simulink model "QuadModel"  (R2022b)
settings: Solver=VariableStepAuto  StartTime=0.0  StopTime=50  RelTol=1e-3  AbsTol=1e-3  EnableMultiTasking=on
undefined symbols (not defined in the file): Ixx, Iyy, Izz, k, mass, prD, prI, prP, X, Y, Z, zD, zI, zP
libraries: sm_lib x42, nesl_utility x35, slpidlib x4
(part 1 of 3)
settings Model: Creator=hrishavdas  LastModifiedBy=sudip
settings SolverCC: AutoScaleAbsTol=off  AlgebraicLoopSolver=TrustRegion  MaxZcPerStep=1
settings DataIOCC: LimitDataPoints=on  MaxDataPoints=10000
settings OptimizationCC: LifeSpan=inf
settings DebuggingCC: UnconnectedInputMsg=warning  UnconnectedOutputMsg=warning  UnconnectedLineMsg=warning  AllowSymbolicDim=off  SFUnexpectedBacktrackingDiag=warning  SFNoUnconditionalDefaultTransitionDiag=warning  SFExecutionAtInitializationDiag=none  SFMachineParentedDataDiag=warning  ArithmeticOperatorsInVariantConditions=warning
settings ModelReferenceCC: EnableRefExpFcnMdlSchedulingChecks=on
settings SFSimCC: SimUseLocalCustomCode=off  CustomCodeUndefinedFunction=UseInterfaceOnly
settings RTWCC: RTWUseLocalCustomCode=off  DLArmComputeVersion=19.05
settings CodeAppCC: StateflowObjectComments=on
settings GRTTargetCC: TargetLangStandard=C89/C90 (ANSI)
settings ConfigComp: CovMetricSettings=dw  CovSaveCumulativeToWorkspaceVar=on  CovSaveSingleToWorkspaceVar=on  CovExternalEMLEnable=off  CovSFcnEnable=off
settings SimscapeCC: SimscapeLogType=all  SimscapeLogSimulationStatistics=on  SimscapeLogDataHistory=10000

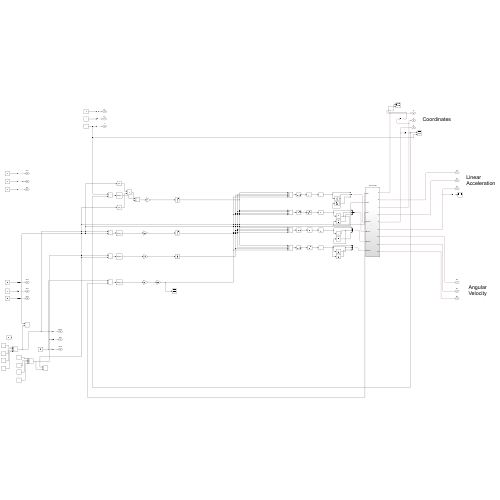
[thumbnail: Simulink's stored preview of the top-level diagram]
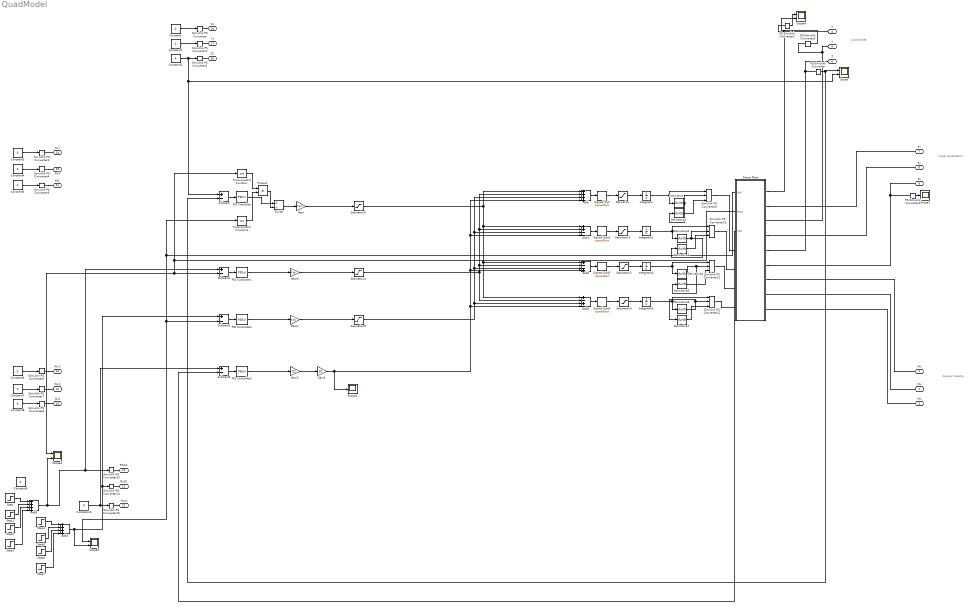
== system QuadModel ==
  note: Coordinates
  note: Linear Acceleration
  note: Angular Velocity
  Add : Sum  Inputs=++++
  Add1 : Sum  Inputs=++--
  Add2 : Sum  Inputs=+--+
  Add3 : Sum  Inputs=+-+-
  Add4 : Sum  Inputs=++++
  Add5 : Sum  Inputs=++++
  Constant{,1,3..9,11} (10 alike) : Constant  Value=0
  Constant2 : Constant  Value=4
  Derivative{,1..7} (8 alike) : Derivative
  Divide : Product  Inputs=*/
  Drone Plant : Subsystem
  Gain : Gain  Gain=mass
  Gain1 : Gain  Gain=Ixx
  Gain2 : Gain  Gain=Izz
  Gain3 : Gain  Gain=10
  Gain6 : Gain  Gain=Iyy
  Integrator{,2,4,6} (4 alike) : Integrator
  PID Controller : slpidlib/PID Controller  Controller=PID  Form=Parallel  TimeDomain=Continuous-time  UseExternalTs=off  SampleTime=-1  IntegratorMethod=Forward Euler  FilterMethod=Forward Euler  ControllerParametersSource=internal  P=zP  I=zI  UseKiTs=off  D=zD  N=100  UseFilter=on  TunerSelectOption=Transfer Function Based (PID Tuner App)  InitialConditionSource=internal  InitialConditionForIntegrator=0  InitialConditionForFilter=0  DifferentiatorICPrevScaledInput=0  ExternalReset=none  TrackingMode=off  Kt=1  LimitOutput=off  SatLimitsSource=internal  UpperSaturationLimit=inf  LowerSaturationLimit=-inf  LinearizeAsGain=on  AntiWindupMode=none  Kb=1  LimitIntegrator=off  UpperIntegratorSaturationLimit=inf  LowerIntegratorSaturationLimit=-inf  POutMin=[]  POutMax=[]  IOutMin=[]  IOutMax=[]  DOutMin=[]  DOutMax=[]  NOutMin=[]  NOutMax=[]  SumOutMin=[]  SumOutMax=[]  SaturationOutMin=[]  SaturationOutMax=[]  PParamMin=[]  PParamMax=[]  IParamMin=[]  IParamMax=[]  DParamMin=[]  DParamMax=[]  NParamMin=[]  NParamMax=[]  KbParamMin=[]  KbParamMax=[]  KtParamMin=[]  KtParamMax=[]  KbOutMin=[]  KbOutMax=[]  KtOutMin=[]  KtOutMax=[]  IntegratorOutMin=[]  IntegratorOutMax=[]  FilterOutMin=[]  FilterOutMax=[]  SumI1OutMin=[]  SumI1OutMax=[]  SumI2OutMin=[]  SumI2OutMax=[]  SumI3OutMin=[]  SumI3OutMax=[]  SumI4OutMin=[]  SumI4OutMax=[]  SumDOutMin=[]  SumDOutMax=[]  DifferentiatorOutMin=[]  DifferentiatorOutMax=[]  FilterDiffOutCoefMin=[]  FilterDiffOutCoefMax=[]  ReciprocalOutMin=[]  ReciprocalOutMax=[]  SumDenOutMin=[]  SumDenOutMax=[]  SumNumOutMin=[]  SumNumOutMax=[]  DivideOutMin=[]  DivideOutMax=[]  UdiffTsProdOutMin=[]  UdiffTsProdOutMax=[]  NTsProdOutMin=[]  NTsProdOutMax=[]  UintegralTsProdOutMin=[]  UintegralTsProdOutMax=[]  UngainTsProdOutMin=[]  UngainTsProdOutMax=[]  ClampingZeroOutDataTypeStr=Inherit: Inherit via back propagation  ClampingZeroOutMin=[]  ClampingZeroOutMax=[]  FilterDenConstantOutDataTypeStr=Inherit: Inherit via back propagation  FilterDenConstantOutMin=[]  FilterDenConstantOutMax=[]  PCopyOutDataTypeStr=Inherit: Inherit via back propagation  PCopyOutMin=[]  PCopyOutMax=[]  NCopyOutDataTypeStr=Inherit: Inherit via back propagation  NCopyOutMin=[]  NCopyOutMax=[]  IntegratorContinuousStateAttributes=''  IntegratorStateMustResolveToSignalObject=off  IntegratorRTWStateStorageClass=Auto  FilterContinuousStateAttributes=''  FilterStateMustResolveToSignalObject=off  FilterRTWStateStorageClass=Auto  ParallelPVariant=InternalParameters  IdealPVariant=Disabled  IVariant=InternalParameters  DVariant=InternalParameters  IntegratorVariant=Continuous  SatVariant=Disabled  AWVariant=Passthrough  PCopyVariant=Disabled  TRVariant=Disabled  FdbkBlocksVariant=Forward  IdealPFdbkVariant=Disabled  SatFdbkVariant=Disabled  DerivativeFilterVariant=ContFilter  NVariant=InternalParameters  NCopyVariant=Disabled  FilterICVariant=InternalICsFilter  IntegratorICVariant=InternalICs  ExternalResetVariant=Disabled  TRSumVariant=Passthrough  SumFdbkVariant=Disabled  SumVariant=Sum_PID  TsampFilterVariant=InternalTs  TsampNgainVariant=Passthrough  TsampIntegralVariant=Passthrough  ExternalSaturationOutDataTypeStr=Inherit: Same as second input
  PID Controller1 : slpidlib/PID Controller  Controller=PID  Form=Parallel  TimeDomain=Continuous-time  UseExternalTs=off  SampleTime=-1  IntegratorMethod=Forward Euler  FilterMethod=Forward Euler  ControllerParametersSource=internal  P=prP  I=prI  UseKiTs=off  D=prD  N=100  UseFilter=on  TunerSelectOption=Transfer Function Based (PID Tuner App)  InitialConditionSource=internal  InitialConditionForIntegrator=0  InitialConditionForFilter=0  DifferentiatorICPrevScaledInput=0  ExternalReset=none  TrackingMode=off  Kt=1  LimitOutput=off  SatLimitsSource=internal  UpperSaturationLimit=inf  LowerSaturationLimit=-inf  LinearizeAsGain=on  AntiWindupMode=none  Kb=1  LimitIntegrator=off  UpperIntegratorSaturationLimit=inf  LowerIntegratorSaturationLimit=-inf  POutMin=[]  POutMax=[]  IOutMin=[]  IOutMax=[]  DOutMin=[]  DOutMax=[]  NOutMin=[]  NOutMax=[]  SumOutMin=[]  SumOutMax=[]  SaturationOutMin=[]  SaturationOutMax=[]  PParamMin=[]  PParamMax=[]  IParamMin=[]  IParamMax=[]  DParamMin=[]  DParamMax=[]  NParamMin=[]  NParamMax=[]  KbParamMin=[]  KbParamMax=[]  KtParamMin=[]  KtParamMax=[]  KbOutMin=[]  KbOutMax=[]  KtOutMin=[]  KtOutMax=[]  IntegratorOutMin=[]  IntegratorOutMax=[]  FilterOutMin=[]  FilterOutMax=[]  SumI1OutMin=[]  SumI1OutMax=[]  SumI2OutMin=[]  SumI2OutMax=[]  SumI3OutMin=[]  SumI3OutMax=[]  SumI4OutMin=[]  SumI4OutMax=[]  SumDOutMin=[]  SumDOutMax=[]  DifferentiatorOutMin=[]  DifferentiatorOutMax=[]  FilterDiffOutCoefMin=[]  FilterDiffOutCoefMax=[]  ReciprocalOutMin=[]  ReciprocalOutMax=[]  SumDenOutMin=[]  SumDenOutMax=[]  SumNumOutMin=[]  SumNumOutMax=[]  DivideOutMin=[]  DivideOutMax=[]  UdiffTsProdOutMin=[]  UdiffTsProdOutMax=[]  NTsProdOutMin=[]  NTsProdOutMax=[]  UintegralTsProdOutMin=[]  UintegralTsProdOutMax=[]  UngainTsProdOutMin=[]  UngainTsProdOutMax=[]  ClampingZeroOutDataTypeStr=Inherit: Inherit via back propagation  ClampingZeroOutMin=[]  ClampingZeroOutMax=[]  FilterDenConstantOutDataTypeStr=Inherit: Inherit via back propagation  FilterDenConstantOutMin=[]  FilterDenConstantOutMax=[]  PCopyOutDataTypeStr=Inherit: Inherit via back propagation  PCopyOutMin=[]  PCopyOutMax=[]  NCopyOutDataTypeStr=Inherit: Inherit via back propagation  NCopyOutMin=[]  NCopyOutMax=[]  IntegratorContinuousStateAttributes=''  IntegratorStateMustResolveToSignalObject=off  IntegratorRTWStateStorageClass=Auto  FilterContinuousStateAttributes=''  FilterStateMustResolveToSignalObject=off  FilterRTWStateStorageClass=Auto  ParallelPVariant=InternalParameters  IdealPVariant=Disabled  IVariant=InternalParameters  DVariant=InternalParameters  IntegratorVariant=Continuous  SatVariant=Disabled  AWVariant=Passthrough  PCopyVariant=Disabled  TRVariant=Disabled  FdbkBlocksVariant=Forward  IdealPFdbkVariant=Disabled  SatFdbkVariant=Disabled  DerivativeFilterVariant=ContFilter  NVariant=InternalParameters  NCopyVariant=Disabled  FilterICVariant=InternalICsFilter  IntegratorICVariant=InternalICs  ExternalResetVariant=Disabled  TRSumVariant=Passthrough  SumFdbkVariant=Disabled  SumVariant=Sum_PID  TsampFilterVariant=InternalTs  TsampNgainVariant=Passthrough  TsampIntegralVariant=Passthrough  ExternalSaturationOutDataTypeStr=Inherit: Same as second input
  PID Controller2 : slpidlib/PID Controller  Controller=PID  Form=Parallel  TimeDomain=Continuous-time  UseExternalTs=off  SampleTime=-1  IntegratorMethod=Forward Euler  FilterMethod=Forward Euler  ControllerParametersSource=internal  P=prP  I=prI  UseKiTs=off  D=prD  N=100  UseFilter=on  TunerSelectOption=Transfer Function Based (PID Tuner App)  InitialConditionSource=internal  InitialConditionForIntegrator=0  InitialConditionForFilter=0  DifferentiatorICPrevScaledInput=0  ExternalReset=none  TrackingMode=off  Kt=1  LimitOutput=off  SatLimitsSource=internal  UpperSaturationLimit=inf  LowerSaturationLimit=-inf  LinearizeAsGain=on  AntiWindupMode=none  Kb=1  LimitIntegrator=off  UpperIntegratorSaturationLimit=inf  LowerIntegratorSaturationLimit=-inf  POutMin=[]  POutMax=[]  IOutMin=[]  IOutMax=[]  DOutMin=[]  DOutMax=[]  NOutMin=[]  NOutMax=[]  SumOutMin=[]  SumOutMax=[]  SaturationOutMin=[]  SaturationOutMax=[]  PParamMin=[]  PParamMax=[]  IParamMin=[]  IParamMax=[]  DParamMin=[]  DParamMax=[]  NParamMin=[]  NParamMax=[]  KbParamMin=[]  KbParamMax=[]  KtParamMin=[]  KtParamMax=[]  KbOutMin=[]  KbOutMax=[]  KtOutMin=[]  KtOutMax=[]  IntegratorOutMin=[]  IntegratorOutMax=[]  FilterOutMin=[]  FilterOutMax=[]  SumI1OutMin=[]  SumI1OutMax=[]  SumI2OutMin=[]  SumI2OutMax=[]  SumI3OutMin=[]  SumI3OutMax=[]  SumI4OutMin=[]  SumI4OutMax=[]  SumDOutMin=[]  SumDOutMax=[]  DifferentiatorOutMin=[]  DifferentiatorOutMax=[]  FilterDiffOutCoefMin=[]  FilterDiffOutCoefMax=[]  ReciprocalOutMin=[]  ReciprocalOutMax=[]  SumDenOutMin=[]  SumDenOutMax=[]  SumNumOutMin=[]  SumNumOutMax=[]  DivideOutMin=[]  DivideOutMax=[]  UdiffTsProdOutMin=[]  UdiffTsProdOutMax=[]  NTsProdOutMin=[]  NTsProdOutMax=[]  UintegralTsProdOutMin=[]  UintegralTsProdOutMax=[]  UngainTsProdOutMin=[]  UngainTsProdOutMax=[]  ClampingZeroOutDataTypeStr=Inherit: Inherit via back propagation  ClampingZeroOutMin=[]  ClampingZeroOutMax=[]  FilterDenConstantOutDataTypeStr=Inherit: Inherit via back propagation  FilterDenConstantOutMin=[]  FilterDenConstantOutMax=[]  PCopyOutDataTypeStr=Inherit: Inherit via back propagation  PCopyOutMin=[]  PCopyOutMax=[]  NCopyOutDataTypeStr=Inherit: Inherit via back propagation  NCopyOutMin=[]  NCopyOutMax=[]  IntegratorContinuousStateAttributes=''  IntegratorStateMustResolveToSignalObject=off  IntegratorRTWStateStorageClass=Auto  FilterContinuousStateAttributes=''  FilterStateMustResolveToSignalObject=off  FilterRTWStateStorageClass=Auto  ParallelPVariant=InternalParameters  IdealPVariant=Disabled  IVariant=InternalParameters  DVariant=InternalParameters  IntegratorVariant=Continuous  SatVariant=Disabled  AWVariant=Passthrough  PCopyVariant=Disabled  TRVariant=Disabled  FdbkBlocksVariant=Forward  IdealPFdbkVariant=Disabled  SatFdbkVariant=Disabled  DerivativeFilterVariant=ContFilter  NVariant=InternalParameters  NCopyVariant=Disabled  FilterICVariant=InternalICsFilter  IntegratorICVariant=InternalICs  ExternalResetVariant=Disabled  TRSumVariant=Passthrough  SumFdbkVariant=Disabled  SumVariant=Sum_PID  TsampFilterVariant=InternalTs  TsampNgainVariant=Passthrough  TsampIntegralVariant=Passthrough  ExternalSaturationOutDataTypeStr=Inherit: Same as second input
  PID Controller3 : slpidlib/PID Controller  Controller=PID  Form=Parallel  TimeDomain=Continuous-time  UseExternalTs=off  SampleTime=-1  IntegratorMethod=Forward Euler  FilterMethod=Forward Euler  ControllerParametersSource=internal  P=1e4  I=5e3  UseKiTs=off  D=1e3  N=100  UseFilter=on  TunerSelectOption=Transfer Function Based (PID Tuner App)  InitialConditionSource=internal  InitialConditionForIntegrator=0  InitialConditionForFilter=0  DifferentiatorICPrevScaledInput=0  ExternalReset=none  TrackingMode=off  Kt=1  LimitOutput=off  SatLimitsSource=internal  UpperSaturationLimit=inf  LowerSaturationLimit=-inf  LinearizeAsGain=on  AntiWindupMode=none  Kb=1  LimitIntegrator=off  UpperIntegratorSaturationLimit=inf  LowerIntegratorSaturationLimit=-inf  POutMin=[]  POutMax=[]  IOutMin=[]  IOutMax=[]  DOutMin=[]  DOutMax=[]  NOutMin=[]  NOutMax=[]  SumOutMin=[]  SumOutMax=[]  SaturationOutMin=[]  SaturationOutMax=[]  PParamMin=[]  PParamMax=[]  IParamMin=[]  IParamMax=[]  DParamMin=[]  DParamMax=[]  NParamMin=[]  NParamMax=[]  KbParamMin=[]  KbParamMax=[]  KtParamMin=[]  KtParamMax=[]  KbOutMin=[]  KbOutMax=[]  KtOutMin=[]  KtOutMax=[]  IntegratorOutMin=[]  IntegratorOutMax=[]  FilterOutMin=[]  FilterOutMax=[]  SumI1OutMin=[]  SumI1OutMax=[]  SumI2OutMin=[]  SumI2OutMax=[]  SumI3OutMin=[]  SumI3OutMax=[]  SumI4OutMin=[]  SumI4OutMax=[]  SumDOutMin=[]  SumDOutMax=[]  DifferentiatorOutMin=[]  DifferentiatorOutMax=[]  FilterDiffOutCoefMin=[]  FilterDiffOutCoefMax=[]  ReciprocalOutMin=[]  ReciprocalOutMax=[]  SumDenOutMin=[]  SumDenOutMax=[]  SumNumOutMin=[]  SumNumOutMax=[]  DivideOutMin=[]  DivideOutMax=[]  UdiffTsProdOutMin=[]  UdiffTsProdOutMax=[]  NTsProdOutMin=[]  NTsProdOutMax=[]  UintegralTsProdOutMin=[]  UintegralTsProdOutMax=[]  UngainTsProdOutMin=[]  UngainTsProdOutMax=[]  ClampingZeroOutDataTypeStr=Inherit: Inherit via back propagation  ClampingZeroOutMin=[]  ClampingZeroOutMax=[]  FilterDenConstantOutDataTypeStr=Inherit: Inherit via back propagation  FilterDenConstantOutMin=[]  FilterDenConstantOutMax=[]  PCopyOutDataTypeStr=Inherit: Inherit via back propagation  PCopyOutMin=[]  PCopyOutMax=[]  NCopyOutDataTypeStr=Inherit: Inherit via back propagation  NCopyOutMin=[]  NCopyOutMax=[]  IntegratorContinuousStateAttributes=''  IntegratorStateMustResolveToSignalObject=off  IntegratorRTWStateStorageClass=Auto  FilterContinuousStateAttributes=''  FilterStateMustResolveToSignalObject=off  FilterRTWStateStorageClass=Auto  ParallelPVariant=InternalParameters  IdealPVariant=Disabled  IVariant=InternalParameters  DVariant=InternalParameters  IntegratorVariant=Continuous  SatVariant=Disabled  AWVariant=Passthrough  PCopyVariant=Disabled  TRVariant=Disabled  FdbkBlocksVariant=Forward  IdealPFdbkVariant=Disabled  SatFdbkVariant=Disabled  DerivativeFilterVariant=ContFilter  NVariant=InternalParameters  NCopyVariant=Disabled  FilterICVariant=InternalICsFilter  IntegratorICVariant=InternalICs  ExternalResetVariant=Disabled  TRSumVariant=Passthrough  SumFdbkVariant=Disabled  SumVariant=Sum_PID  TsampFilterVariant=InternalTs  TsampNgainVariant=Passthrough  TsampIntegralVariant=Passthrough  ExternalSaturationOutDataTypeStr=Inherit: Same as second input
  PS-Simulink Converter{,1..3} (4 alike) : nesl_utility/PS-Simulink Converter  PhysicalDomain=network_engine_domain  SubClassName=ps_output  LeftPortType=input  RightPortType=output  PseudoPeriodic=off  Frequencies=[]  VectorFormat=inherit  Unit=inherit  AffineConversion=off
  Product : Product
  Saturation{,1..3} (4 alike) : Saturate  UpperLimit=225  LowerLimit=-225
  Saturation4 : Saturate  UpperLimit=1200  LowerLimit=-1200
  Saturation5 : Saturate  UpperLimit=1200  LowerLimit=-1200
  Saturation6 : Saturate  UpperLimit=15000  LowerLimit=-15000
  Scope{,3..5} (4 alike) : Scope  NumInputPorts=2
  Scope1 : Scope
  Scope2 : Scope
  Signed Sqrt{,1..3} (4 alike) : Sqrt  Operator=signedSqrt
  Simulink-PS Converter{,1..8,13..15} (12 alike) : nesl_utility/Simulink-PS Converter  PhysicalDomain=network_engine_domain  SubClassName=ps_input  LeftPortType=input  RightPortType=output  PseudoPeriodic=off  Frequencies=[]  NoiseDistribution=none  NoiseParameters=[]  Unit=1  AffineConversion=off  FilteringAndDerivatives=provide  SimscapeFilterOrder=1  InputFilterTimeConstant=0.001  UdotUserProvided=0
  Simulink-PS Converter{9..12} (4 alike) : nesl_utility/Simulink-PS Converter  PhysicalDomain=network_engine_domain  SubClassName=ps_input  LeftPortType=input  RightPortType=output  PseudoPeriodic=off  Frequencies=[]  NoiseDistribution=none  NoiseParameters=[]  Unit=1  AffineConversion=off  FilteringAndDerivatives=provide  SimscapeFilterOrder=1  InputFilterTimeConstant=0.001  UdotUserProvided=2
  Step : Step  Time=10  After=5  SampleTime=0
  Step1 : Step  Time=10.1  After=-5  SampleTime=0
  Step2 : Step  Time=20  After=-3.7  SampleTime=0
  Step3 : Step  Time=20.1  After=3.7  SampleTime=0
  Step4 : Step  Time=30  After=5  SampleTime=0
  Step5 : Step  Time=30.1  After=-5  SampleTime=0
  Step6 : Step  Time=40  After=-3.7  SampleTime=0
  Step7 : Step  Time=40.1  After=3.7  SampleTime=0
  Subtract{,1..3} (4 alike) : Sum  Inputs=+-
  Trigonometric Function : Trigonometry  Operator=cos
  Trigonometric Function1 : Trigonometry  Operator=cos
  Wx : PMIOPort  Side=Left
  Wy : PMIOPort  Port=2  Side=Left
  Wz : PMIOPort  Port=3  Side=Left
  X : PMIOPort  Port=4  Side=Left
  Y : PMIOPort  Port=5  Side=Left
  Z : PMIOPort  Port=6  Side=Left
  ax : PMIOPort  Port=7  Side=Left
  ay : PMIOPort  Port=8  Side=Left
  az : PMIOPort  Port=9  Side=Left
  Pitch1 : PMIOPort  Port=10  Side=Left
  Roll1 : PMIOPort  Port=11  Side=Left
  Yaw1 : PMIOPort  Port=12  Side=Left
  Wx1 : PMIOPort  Port=13  Side=Left
  Wy1 : PMIOPort  Port=14  Side=Left
  Wz1 : PMIOPort  Port=15  Side=Left
  X1 : PMIOPort  Port=16  Side=Left
  Y1 : PMIOPort  Port=17  Side=Left
  Z1 : PMIOPort  Port=18  Side=Left
  ax1 : PMIOPort  Port=19  Side=Left
  ay1 : PMIOPort  Port=20  Side=Left
  az1 : PMIOPort  Port=21  Side=Left
  wires:
  Constant/1 -> Simulink-PS Converter/1
  Constant1/1 -> Simulink-PS Converter1/1
  Constant3/1 -> Simulink-PS Converter3/1
  Constant4/1 -> Simulink-PS Converter4/1
  Constant5/1 -> Simulink-PS Converter5/1
  Constant8/1 -> Simulink-PS Converter8/1
  Constant7/1 -> Simulink-PS Converter7/1
  Constant6/1 -> Simulink-PS Converter6/1
  Derivative/1 -> Derivative1/1, Simulink-PS Converter9/2
  Derivative1/1 -> Simulink-PS Converter9/3
  Integrator/1 -> Simulink-PS Converter9/1, Derivative/1
  Integrator2/1 -> Derivative2/1, Simulink-PS Converter10/1
  Derivative3/1 -> Simulink-PS Converter10/3
  Derivative2/1 -> Derivative3/1, Simulink-PS Converter10/2
  Derivative4/1 -> Derivative5/1, Simulink-PS Converter11/2
  Derivative5/1 -> Simulink-PS Converter11/3
  Integrator4/1 -> Simulink-PS Converter11/1, Derivative4/1
  Integrator6/1 -> Derivative6/1, Simulink-PS Converter12/1
  Derivative7/1 -> Simulink-PS Converter12/3
  Derivative6/1 -> Derivative7/1, Simulink-PS Converter12/2
  PS-Simulink Converter/1 -> Subtract/2, Scope/1
  Constant2/1 -> Simulink-PS Converter2/1, Subtract/1, Scope/2
  Subtract/1 -> PID Controller/1
  Trigonometric Function/1 -> Product/1
  Trigonometric Function1/1 -> Product/2
  PID Controller/1 -> Divide/1
  Product/1 -> Divide/2
  Divide/1 -> Gain/1
  PS-Simulink Converter1/1 -> Scope1/1
  Add/1 -> Signed Sqrt/1
  Add2/1 -> Signed Sqrt2/1
  Add1/1 -> Signed Sqrt1/1
  Add3/1 -> Signed Sqrt3/1
  PID Controller1/1 -> Gain6/1
  Subtract1/1 -> PID Controller1/1
  Subtract2/1 -> PID Controller2/1
  PID Controller2/1 -> Gain1/1
  Drone Plant/2(Pitch) -> Scope3/1, Subtract1/2, Trigonometric Function/1
  Drone Plant/1(Roll) -> Scope5/1, Subtract2/2, Trigonometric Function1/1
  Gain6/1 -> Saturation4/1
  Signed Sqrt3/1 -> Saturation3/1
  Saturation3/1 -> Integrator6/1
  Saturation2/1 -> Integrator4/1
  Signed Sqrt2/1 -> Saturation2/1
  Signed Sqrt1/1 -> Saturation1/1
  Saturation1/1 -> Integrator2/1
  Signed Sqrt/1 -> Saturation/1
  Saturation/1 -> Integrator/1
  Saturation4/1 -> Add3/2, Add/2, Add1/2, Add2/2
  Gain1/1 -> Saturation5/1
  Saturation5/1 -> Add3/3, Add1/3, Add/3, Add2/3
  Gain/1 -> Saturation6/1
  Saturation6/1 -> Add3/1, Add2/1, Add1/1, Add/1
  Subtract3/1 -> PID Controller3/1
  PID Controller3/1 -> Gain2/1
  Drone Plant/3(Yaw) -> Subtract3/2
  Constant11/1 -> Subtract3/1, Simulink-PS Converter15/1
  Step/1 -> Add5/1
  Step1/1 -> Add5/2
  Gain2/1 -> Gain3/1
  Gain3/1 -> Scope2/1, Add/4, Add1/4, Add2/4, Add3/4
  Add5/1 -> Scope3/2, Subtract1/1, Simulink-PS Converter13/1
  Step2/1 -> Add5/3
  Step3/1 -> Add5/4
  PS-Simulink Converter2/1 -> Scope4/1
  Step7/1 -> Add4/4
  Step6/1 -> Add4/3
  Step5/1 -> Add4/2
  Step4/1 -> Add4/1
  Add4/1 -> Scope5/2, Subtract2/1, Simulink-PS Converter14/1
  PS-Simulink Converter3/1 -> Scope4/2
  connections:
  Drone Plant/LConn1 -- PS-Simulink Converter2/LConn1 -- X/RConn1
  Drone Plant/LConn2 -- ax/RConn1
  Y/RConn1 -- PS-Simulink Converter3/LConn1 -- Drone Plant/LConn3
  Drone Plant/LConn4 -- ay/RConn1
  Drone Plant/LConn5 -- PS-Simulink Converter/LConn1 -- Z/RConn1
  Drone Plant/LConn6 -- PS-Simulink Converter1/LConn1 -- az/RConn1
  Drone Plant/LConn7 -- Wx/RConn1
  Wy/RConn1 -- Drone Plant/LConn8
  Wz/RConn1 -- Drone Plant/LConn9
  Simulink-PS Converter/RConn1 -- X1/RConn1
  Y1/RConn1 -- Simulink-PS Converter1/RConn1
  Z1/RConn1 -- Simulink-PS Converter2/RConn1
  ax1/RConn1 -- Simulink-PS Converter3/RConn1
  Simulink-PS Converter4/RConn1 -- ay1/RConn1
  Simulink-PS Converter5/RConn1 -- az1/RConn1
  Simulink-PS Converter8/RConn1 -- Wz1/RConn1
  Simulink-PS Converter6/RConn1 -- Wx1/RConn1
  Simulink-PS Converter7/RConn1 -- Wy1/RConn1
  Simulink-PS Converter9/RConn1 -- Drone Plant/RConn1
  Simulink-PS Converter10/RConn1 -- Drone Plant/RConn2
  Simulink-PS Converter11/RConn1 -- Drone Plant/RConn3
  Simulink-PS Converter12/RConn1 -- Drone Plant/RConn4
  Simulink-PS Converter13/RConn1 -- Pitch1/RConn1
  Simulink-PS Converter14/RConn1 -- Roll1/RConn1
  Simulink-PS Converter15/RConn1 -- Yaw1/RConn1
